simulink model "SystemSISOC"  (R2023b)
settings: Solver=ode45  StartTime=0.0  StopTime=tend  MaxStep=0.01  RelTol=1e-3  EnableMultiTasking=on
InitFcn:
  | PIV_n1 = zeros(3,3);
  | phat_RIV_n1 = zeros(3,1);
values from neighbouring files (symbols this model uses):
  sigma2e = 0.1    [zad3.m]
  TF = 8*Tp    (= 0.4)    [zad3.m]
  Tp = 0.05    [zad3.m]
libraries: simulink x1
settings Model: Creator=kszygenda  LastModifiedBy=Rafał
settings SolverCC: AlgebraicLoopSolver=TrustRegion
settings DataIOCC: LimitDataPoints=on  SaveFormat=Array  SignalLoggingSaveFormat=ModelDataLogs  ReturnWorkspaceOutputs=off
settings OptimizationCC: InitFltsAndDblsToZero=on  LifeSpan=inf
settings DebuggingCC: SaveWithParameterizedLinksMsg=none  UnderspecifiedInitializationDetection=Classic  MergeDetectMultiDrivingBlocksExec=none  SignalResolutionControl=TryResolveAllWithWarning  SolverPrmCheckMsg=warning  MultiTaskDSMMsg=warning  MultiTaskCondExecSysMsg=none  FcnCallInpInsideContextMsg=warning  UnconnectedInputMsg=warning  UnconnectedOutputMsg=warning  UnconnectedLineMsg=warning  SFUnexpectedBacktrackingDiag=warning  SFNoUnconditionalDefaultTransitionDiag=warning  SFExecutionAtInitializationDiag=none  UnderSpecifiedDimensionMsg=warning  ArithmeticOperatorsInVariantConditions=warning
settings HardwareCC: ProdBitPerPointer=32  ProdBitPerSizeT=32  ProdBitPerPtrDiffT=32  ProdLargestAtomicFloat=None  ProdIntDivRoundTo=Undefined  ProdEndianess=Unspecified  ProdWordSize=32  ProdHWDeviceType=32-bit Generic
settings ModelReferenceCC: PropagateSignalLabelsOutOfModel=off
settings CodeAppCC: StateflowObjectComments=on
settings GRTTargetCC: TargetFcnLib=ansi_tfl_tmw.mat  TargetLangStandard=C89/C90 (ANSI)  CombineOutputUpdateFcns=off  GRTInterface=on
settings ConfigComp: CovMetricSettings=dw  CovSaveCumulativeToWorkspaceVar=on  CovSaveSingleToWorkspaceVar=on

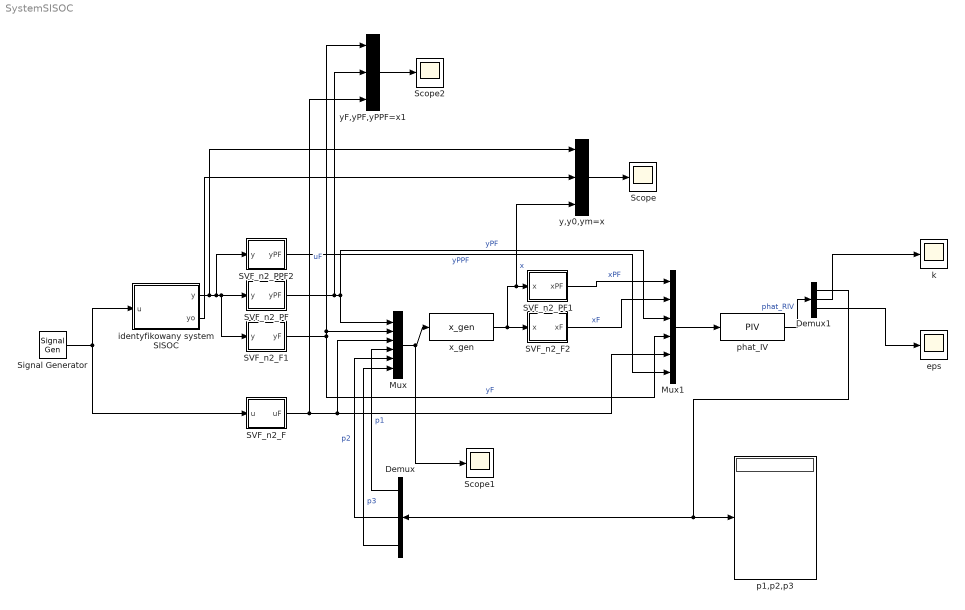
== system SystemSISOC ==
  Demux : Demux  Outputs=3
  Demux1 : Demux  Outputs=[3;3;1]
  Mux : Mux  Inputs=6
  Mux1 : Mux  Inputs=6
  SVF_n2_F : Subsystem
  SVF_n2_F1 : Subsystem
  SVF_n2_F2 : Subsystem
  SVF_n2_PF : Subsystem
  SVF_n2_PF1 : Subsystem
  SVF_n2_PPF2 : Subsystem
  Scope : Scope
  Scope1 : Scope
  Scope2 : Scope
  Signal Generator : SignalGenerator  WaveForm=square  Frequency=0.04
  eps : Scope
  identyfikowany system SISOC : Subsystem
  k : Scope
  p1,p2,p3 : Display
  phat_IV : MATLABFcn  MATLABFcn=PIV  OutputDimensions=7  OutputSignalType=real
  x_gen : MATLABFcn  MATLABFcn=x_gen  OutputDimensions=1
  y,y0,ym=x : Mux  Inputs=3
  yF,yPF,yPPF=x1 : Mux  Inputs=3
  wires:
  Signal Generator/1 -> SVF_n2_F/1(u), identyfikowany system SISOC/1(u)
  identyfikowany system SISOC/1(y) -> y,y0,ym=x/1, SVF_n2_PPF2/1(y), SVF_n2_PF/1(y), SVF_n2_F1/1(y)
  x_gen/1 -> y,y0,ym=x/3, SVF_n2_PF1/1(x), SVF_n2_F2/1(x)  "x"
  phat_IV/1 -> Demux1/1  "phat_RIV"
  Mux/1 -> Scope1/1, x_gen/1
  SVF_n2_F/1(uF) -> Mux1/5, Mux/3, yF,yPF,yPPF=x1/3  "uF"
  SVF_n2_F1/1(yF) -> Mux/2, yF,yPF,yPPF=x1/1, Mux1/4  "yF"
  SVF_n2_PF/1(yPF) -> Mux1/3, Mux/1, yF,yPF,yPPF=x1/2  "yPF"
  SVF_n2_PF1/1(xPF) -> Mux1/1  "xPF"
  SVF_n2_F2/1(xF) -> Mux1/2  "xF"
  Mux1/1 -> phat_IV/1
  y,y0,ym=x/1 -> Scope/1
  identyfikowany system SISOC/2(yo) -> y,y0,ym=x/2
  SVF_n2_PPF2/1(yPF) -> Mux1/6  "yPPF"
  Demux/1 -> Mux/4  "p1"
  Demux/2 -> Mux/5  "p2"
  Demux/3 -> Mux/6  "p3"
  yF,yPF,yPPF=x1/1 -> Scope2/1
  Demux1/1 -> Demux/1, p1,p2,p3/1
  Demux1/2 -> k/1
  Demux1/3 -> eps/1

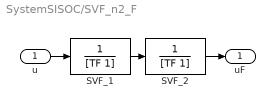
== system SystemSISOC/SVF_n2_F ==
  u : Inport
  SVF_1 : TransferFcn  Denominator=[TF 1]
  SVF_2 : TransferFcn  Denominator=[TF 1]
  uF : Outport
  wires:
  SVF_1/1 -> SVF_2/1
  u/1 -> SVF_1/1
  SVF_2/1 -> uF/1

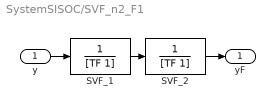
== system SystemSISOC/SVF_n2_F1 ==
  y : Inport
  SVF_1 : TransferFcn  Denominator=[TF 1]
  SVF_2 : TransferFcn  Denominator=[TF 1]
  yF : Outport
  wires:
  SVF_1/1 -> SVF_2/1
  y/1 -> SVF_1/1
  SVF_2/1 -> yF/1

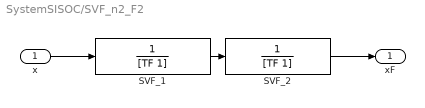
== system SystemSISOC/SVF_n2_F2 ==
  x : Inport
  SVF_1 : TransferFcn  Denominator=[TF 1]
  SVF_2 : TransferFcn  Denominator=[TF 1]
  xF : Outport
  wires:
  SVF_1/1 -> SVF_2/1
  x/1 -> SVF_1/1
  SVF_2/1 -> xF/1

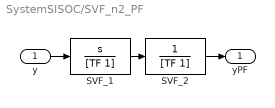
== system SystemSISOC/SVF_n2_PF ==
  y : Inport
  SVF_1 : TransferFcn  Numerator=[1 0]  Denominator=[TF 1]
  SVF_2 : TransferFcn  Denominator=[TF 1]
  yPF : Outport
  wires:
  SVF_1/1 -> SVF_2/1
  y/1 -> SVF_1/1
  SVF_2/1 -> yPF/1

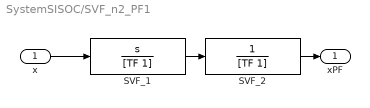
== system SystemSISOC/SVF_n2_PF1 ==
  x : Inport
  SVF_1 : TransferFcn  Numerator=[1 0]  Denominator=[TF 1]
  SVF_2 : TransferFcn  Denominator=[TF 1]
  xPF : Outport
  wires:
  SVF_1/1 -> SVF_2/1
  x/1 -> SVF_1/1
  SVF_2/1 -> xPF/1

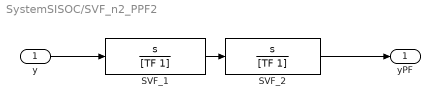
== system SystemSISOC/SVF_n2_PPF2 ==
  y : Inport
  SVF_1 : TransferFcn  Numerator=[1 0]  Denominator=[TF 1]
  SVF_2 : TransferFcn  Numerator=[1 0]  Denominator=[TF 1]
  yPF : Outport
  wires:
  SVF_1/1 -> SVF_2/1
  y/1 -> SVF_1/1
  SVF_2/1 -> yPF/1

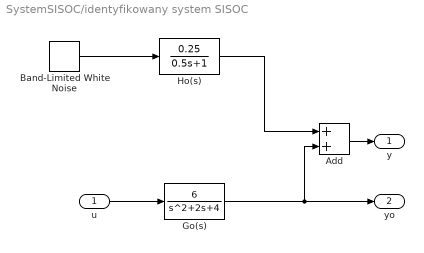
== system SystemSISOC/identyfikowany system SISOC ==
  u : Inport
  Add : Sum
  Band-Limited White Noise : simulink/Sources/Band-Limited White Noise  Cov=[sigma2e]  Ts=Tp*0.1  seed=[2941]
  Go(s) : TransferFcn  Numerator=[6]  Denominator=[1 2 4]
  Ho(s) : TransferFcn  Numerator=[0.25]  Denominator=[0.5 1]
  y : Outport
  yo : Outport  Port=2
  wires:
  Band-Limited White Noise/1 -> Ho(s)/1
  Ho(s)/1 -> Add/1
  Go(s)/1 -> Add/2, yo/1
  Add/1 -> y/1
  u/1 -> Go(s)/1
